simulink model "mStateSpaceVsMcad"  (R2021b)
settings: Solver=VariableStepAuto  StartTime=0.0  StopTime=1000  RelTol=1e-3  AbsTol=1e-3
model workspace (MATLAB code in the model file + MAT data in the model file):
  TnodesInit = 25*ones(50,1)
  lossEachTypeVal = 20*ones(16,1)
  Amat = 3*eye(50) + ones(50)
  Bmat = eye(50)
  TwindingRef = 20
  statorCopperTempCoeff = 1e-5    (= 1e-05)
  lossDistrEachType = ones(16,50)
  CapMat = ones(50,1)
  CoolantNodeIdxs = [2,4,5]
  AdjacencyMat = [0 0 0 0 0 0 0 0 0 0 0 0 ... (22500 elements, 150x150)]
  CoolantArrayIdxs = [21; 26]
  Friction_Loss_Mat = [0 0 0 0 0 0 0 0 0 0 0 0 ... (600 elements, 60x10)]
  InletCoolIdxs = 26
  Iron_Loss_Rotor_Back_Iron_Mat = [5.88721488028e-06 1.56097290893e-05 2.53322432983e-05 3.50547575073e-05 4.22932634361e-05 4.83272215068e-05 5.43611795774e-05 6.0395137648e-05 6.64290957187e-05 7.24630537893e-05 7.84507163281e-05 8.35639993023e-05 ... (600 elements, 60x10)]
  Iron_Loss_Rotor_Pole_Mat = [0 0 0 0 0 0 0 0 0 0 0 0 ... (600 elements, 60x10)]
  Iron_Loss_Rotor_Tooth_Mat = [0.0278606638652 0.0738715035935 0.119882343322 0.16589318305 0.184288576483 0.189292659205 0.194296741928 0.19930082465 0.204304907373 0.209308990095 0.214192013795 0.216788606579 ... (600 elements, 60x10)]
  Iron_Loss_Stator_Back_Iron_Mat = [0.538257512426 1.42720259745 2.31614768248 3.2050927675 3.70144029641 4.00740901333 4.31337773026 4.61934644718 4.9253151641 5.23128388103 5.53405994351 5.77653662762 ... (600 elements, 60x10)]
  Iron_Loss_Stator_Tooth_Mat = [0.271379868831 0.719570446697 1.16776102456 1.61595160243 1.84620127177 1.97076681088 2.09533234999 2.2198978891 2.34446342821 2.46902896732 2.59210855121 2.687123032 ... (600 elements, 60x10)]
  LossDistrForEachType = [0 0 0 0 0 0 0 0 0 0 0 0 ... (2400 elements, 16x150)]
  Magnet_Loss_Mat = [0 0 0 0 0 0 0 0 0 0 0 0 ... (600 elements, 60x10)]
  OutletCoolIdxs = 21
  RotorCopperTempCoefResistivity = 0.00393
  Rotor_Cage_Loss_Mat = [0.452081247683 6.23621443388 12.0203476201 17.8044808063 27.0746990775 38.0353933249 48.9960875724 59.9567818198 70.9174760673 81.8781703148 93.2562227653 112.516882212 ... (600 elements, 60x10)]
  ShaftTorqueVec = [0.50751379462 6.70424518063 12.9009765666 19.0977079526 25.2944393387 31.4911707247 37.6879021107 43.8846334967 50.0813648827 56.2780962687 62.4748276547 68.6715590407 ... (60 elements, 1x60)]
  SpeedVec = [200 1511.11111111 2822.22222222 4133.33333333 5444.44444444 6755.55555556 8066.66666667 9377.77777778 10688.8888889 12000]
  StateSpaceND : object (value not decoded)
  StatorCopperTempCoefResistivity = 0.00393
  Stator_Copper_Loss_Mat = [2.8235353719 37.2375386139 71.6515418559 106.065545098 145.96632659 188.527762252 231.089197915 273.650633577 316.212069239 358.773504901 402.558474022 469.452209983 ... (600 elements, 60x10)]
  Stray_Load_Loss_Mat = [0.107367111702 1.41831699713 2.72926688255 4.04021676798 5.3511666534 6.66211653882 7.97306642425 9.28401630967 10.5949661951 11.9059160805 13.2168659659 14.5278158514 ... (600 elements, 60x10)]
  Stray_Loss_Stator_Iron_Proportion = 0.95
  TrefRotor = 140
  TrefStator = 100
  TrotorRef = 140
  Windage_Loss_Mat = [0 0 0 0 0 0 0 0 0 0 0 0 ... (600 elements, 60x10)]
  rotorCopperTempCoeff = 0.00393
  speedVal = 4000
  torqueVal = 30
libraries: mcadROM_lib x2
(part 2 of 2)

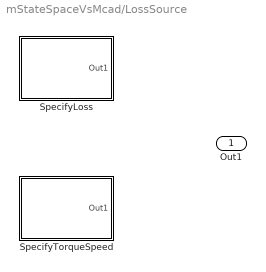
== system mStateSpaceVsMcad/LossSource ==
  SpecifyLoss : Subsystem  VariantControl=SpecifyLoss
  SpecifyTorqueSpeed : Subsystem  VariantControl=SpecifyTorqueSpeed
  Out1 : Outport

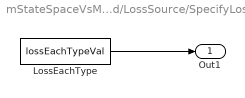
== system mStateSpaceVsMcad/LossSource/SpecifyLoss ==
  LossEachType : Constant  Value=lossEachTypeVal
  Out1 : Outport
  wires:
  LossEachType/1 -> Out1/1

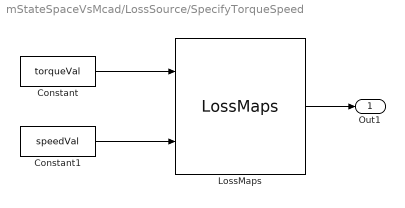
== system mStateSpaceVsMcad/LossSource/SpecifyTorqueSpeed ==
  Constant : Constant  Value=torqueVal
  Constant1 : Constant  Value=speedVal
  LossMaps : mcadROM_lib/LossMaps  ShaftTorqueVec=ShaftTorqueVec  SpeedVec=SpeedVec  Stator_Copper_Loss_Mat=Stator_Copper_Loss_Mat  Rotor_Cage_Loss_Mat=Rotor_Cage_Loss_Mat  Iron_Loss_Stator_Back_Iron_Mat=Iron_Loss_Stator_Back_Iron_Mat  Iron_Loss_Stator_Tooth_Mat=Iron_Loss_Stator_Tooth_Mat  Stray_Loss_Stator_Iron_Proportion=Stray_Loss_Stator_Iron_Proportion  Stray_Load_Loss_Mat=Stray_Load_Loss_Mat  Magnet_Loss_Mat=Magnet_Loss_Mat  Iron_Loss_Rotor_Pole_Mat=Iron_Loss_Rotor_Pole_Mat  Iron_Loss_Rotor_Back_Iron_Mat=Iron_Loss_Rotor_Back_Iron_Mat  Iron_Loss_Rotor_Tooth_Mat=Iron_Loss_Rotor_Tooth_Mat  Friction_Loss_Mat=Friction_Loss_Mat  Windage_Loss_Mat=Windage_Loss_Mat
  Out1 : Outport
  wires:
  LossMaps/1 -> Out1/1
  Constant/1 -> LossMaps/1
  Constant1/1 -> LossMaps/2
